simulink model "TrafficLight"  (R2020a)
settings: Solver=VariableStepAuto  StartTime=0.0  StopTime=100  RelTol=1e-3
settings Model: Creator=Admin  LastModifiedBy=Admin

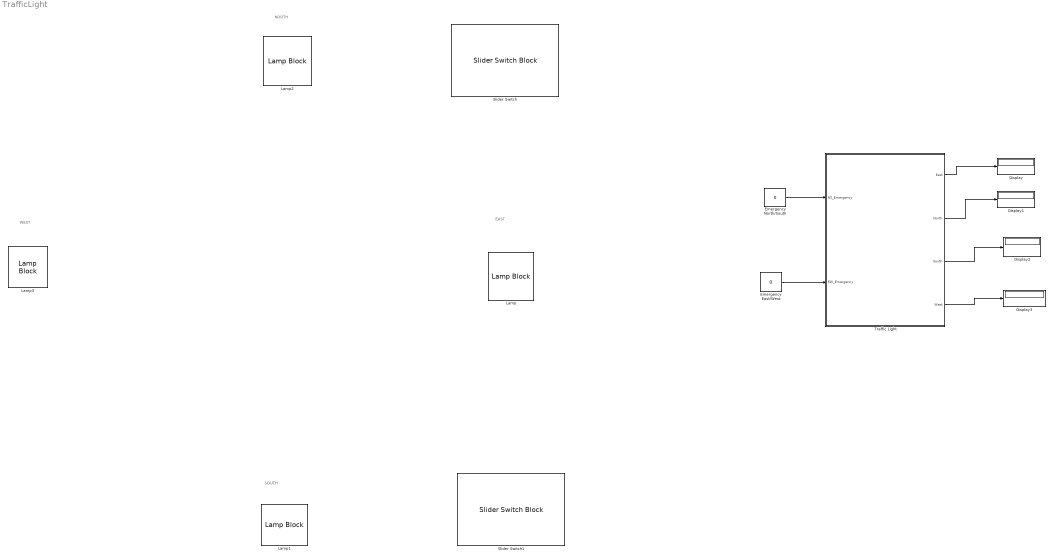
== system TrafficLight ==
  note: NORTH
  note: EAST
  note: SOUTH
  note: WEST
  Display{,1..3} (4 alike) : Display
  Emergency East/West : Constant  Value=0
  Emergency North/South : Constant  Value=0
  Lamp{,1..3} (4 alike) : LampBlock
  Slider Switch : SliderSwitchBlock
      settings: Values={{'Off', 'On'}, [0 1]}
  Slider Switch1 : SliderSwitchBlock
      settings: Values={{'Off', 'On'}, [0 1]}
  Traffic Light : Stateflow chart  TreatAsAtomicUnit=on
  wires:
  Traffic Light/1(East) -> Display/1
  Traffic Light/2(North) -> Display1/1
  Traffic Light/3(South) -> Display2/1
  Traffic Light/4(West) -> Display3/1
  Emergency North/South/1 -> Traffic Light/1(NS_Emergency)
  Emergency East/West/1 -> Traffic Light/2(EW_Emergency)

== stateflow chart TrafficLight/Traffic Light ==
  settings: stateMachineType=MOORE_MACHINE
  state EastWestWait
    East = YELLOW;
    West = YELLOW;
    North = RED;
    South = RED
  state PedestrianGo1
    East = RED;
    West = RED;
    North = RED;
    South = RED
  state EastWestGo
    East = GREEN;
    West = GREEN;
    North = RED;
    South = RED;
  state NorthSouthGo
    East = RED;
    West = RED;
    North = GREEN;
    South = GREEN
  state NorthSouthWait
    East = RED;
    West = RED;
    North = YELLOW;
    South = YELLOW
  state PedestrianGo2
    East = RED;
    West = RED;
    North = RED;
    South = RED
  EastWestWait -> PedestrianGo1 [order 2] : after(2,sec)
  EastWestGo -> EastWestWait [order 2] : after(7,sec)
  PedestrianGo1 -> NorthSouthGo : after(2,sec)
  EastWestWait -> NorthSouthGo [order 1] : after(1,sec)[NS_Emergency == 1]
  (default) -> EastWestGo
  EastWestGo -> NorthSouthGo [order 1] : [NS_Emergency == 1]
  NorthSouthGo -> EastWestGo [order 1] : [EW_Emergency == 1]
  NorthSouthGo -> NorthSouthWait [order 2] : after(7,sec)
  PedestrianGo2 -> EastWestGo : after(2,sec)
  NorthSouthWait -> EastWestGo [order 1] : after(1,sec)[EW_Emergency == 1]
  NorthSouthWait -> PedestrianGo2 [order 2] : after(2,sec)
  data: GREEN constant double =3; RED constant double =1; YELLOW constant double =2; East output; North output; South output; West output; NS_Emergency input; EW_Emergency input
